simulink model "raised_cosine_filter"  (R2026a)
settings: Solver=VariableStepAuto
libraries: dsphdlsigops2 x2, simulink x1, hdlsllib x1

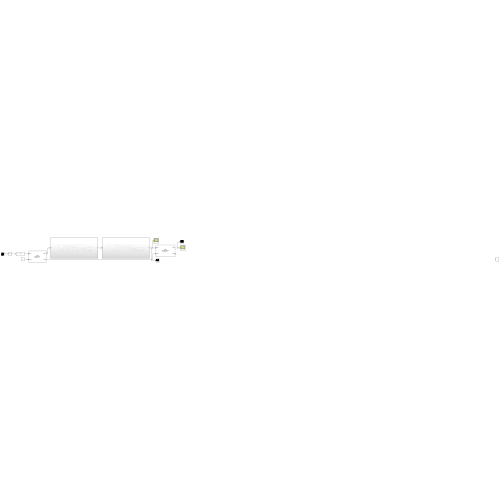
[thumbnail: Simulink's stored preview of the top-level diagram]
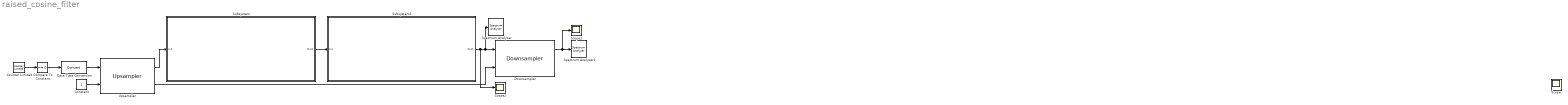
== system raised_cosine_filter ==
  Compare To Constant : simulink/Logic and Bit Operations/Compare To Constant  relop===  const=0  OutDataTypeStr=boolean
  Constant : Constant  OutDataTypeStr=boolean
  Counter Limited : hdlsllib/Sources/Counter Limited  uplimit=1000  tsamp=-1
  Data Type Conversion : DataTypeConversion  SaturateOnIntegerOverflow=off  RndMeth=Floor
  Downsampler : dsphdlsigops2/Downsampler  DownsampleFactor=4  SampleOffset=0  SimulateUsing=Code generation  ResetInputPort=off
  Scope : Scope
      settings: DataLoggingVariableName=ScopeData2  DataLoggingSaveFormat=Array
  Scope1 : Scope
      settings: ActiveDisplayYMinimum=-0.066624588581400856  ActiveDisplayYMaximum=0.22900316407454813  DataLoggingSaveFormat=Array
  Scope2 : Scope
      settings: ActiveDisplayYMinimum=-0.0763979925  ActiveDisplayYMaximum=0.2506889325  DataLoggingSaveFormat=Array
  Spectrum Analyzer : SpectrumAnalyzer  WindowPosition=[269.000000,92.000000,666.000000,500.000000,]  ScopeFrameLocation=window  WindowInvariantSamplesPerUpdate=on  YLimits=[-113.5521 -5.3787]
  Spectrum Analyzer1 : SpectrumAnalyzer  WindowPosition=[339.000000,58.000000,818.000000,500.000000,]  ScopeFrameLocation=window  WindowInvariantSamplesPerUpdate=on  YLimits=[-101.5109 6.6625]
  Subsystem : Subsystem
  Subsystem1 : Subsystem
  Upsampler : dsphdlsigops2/Upsampler  UpsampleFactor=4  SampleOffset=0  NumCycles=1  SimulateUsing=Code generation  ResetInputPort=off  ReadyPort=off
  wires:
  Downsampler/1 -> Scope1/1, Spectrum Analyzer1/1
  Subsystem1/1(Out1) -> Downsampler/1, Spectrum Analyzer/1, Scope2/1
  Upsampler/2 -> Downsampler/2
  Subsystem/1(Out1) -> Subsystem1/1(In1)
  Upsampler/1 -> Subsystem/1(In1)
  Constant/1 -> Upsampler/2
  Data Type Conversion/1 -> Upsampler/1
  Compare To Constant/1 -> Data Type Conversion/1
  Counter Limited/1 -> Compare To Constant/1

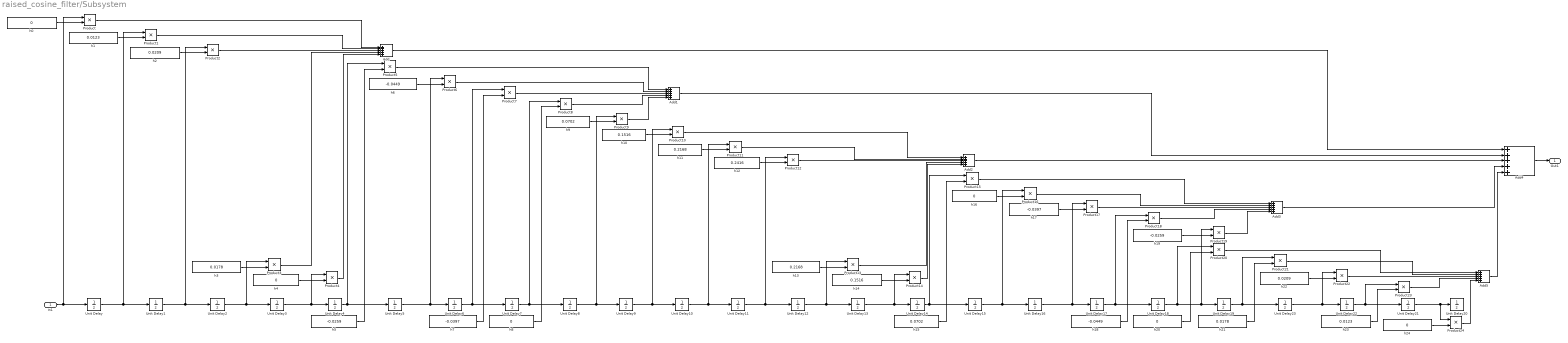
== system raised_cosine_filter/Subsystem ==
  In1 : Inport
  Add{,1..5} (6 alike) : Sum  Inputs=+++++
  Product{,1..24} (25 alike) : Product
  Unit Delay{,1..23} (24 alike) : UnitDelay  SampleTime=-1
  h{0,4,8,16,20,24} (6 alike) : Constant  Value=0
  h1 : Constant  Value=0.0123
  h10 : Constant  Value=0.1516
  h11 : Constant  Value=0.2168
  h12 : Constant  Value=0.2416
  h13 : Constant  Value=0.2168
  h14 : Constant  Value=0.1516
  h15 : Constant  Value=0.0702
  h17 : Constant  Value=-0.0397
  h18 : Constant  Value=-0.0449
  h19 : Constant  Value=-0.0259
  h2 : Constant  Value=0.0209
  h21 : Constant  Value=0.0178
  h22 : Constant  Value=0.0209
  h23 : Constant  Value=0.0123
  h3 : Constant  Value=0.0178
  h5 : Constant  Value=-0.0259
  h6 : Constant  Value=-0.0449
  h7 : Constant  Value=-0.0397
  h9 : Constant  Value=0.0702
  Out1 : Outport
  wires:
  Add4/1 -> Out1/1
  Add5/1 -> Add4/5
  Product24/1 -> Add5/5
  h24/1 -> Product24/2
  Unit Delay21/1 -> Product24/1, Unit Delay20/1
  Product23/1 -> Add5/4
  h23/1 -> Product23/2
  Unit Delay22/1 -> Unit Delay21/1, Product23/1
  Product22/1 -> Add5/3
  Unit Delay23/1 -> Product22/1, Unit Delay22/1
  h22/1 -> Product22/2
  Product21/1 -> Add5/2
  Product20/1 -> Add5/1
  Product19/1 -> Add3/5
  h20/1 -> Product20/2
  Unit Delay18/1 -> Product19/1, Unit Delay19/1, Product20/1
  Product18/1 -> Add3/4
  h19/1 -> Product19/2
  h9/1 -> Product9/2
  h8/1 -> Product8/2
  Product13/1 -> Add2/4
  Product6/1 -> Add1/2
  Unit Delay19/1 -> Product21/1, Unit Delay23/1
  h7/1 -> Product7/2
  Unit Delay6/1 -> Unit Delay7/1, Product7/1
  h12/1 -> Product12/2
  h6/1 -> Product6/2
  Unit Delay/1 -> Product1/1, Unit Delay1/1
  Unit Delay4/1 -> Product5/1, Unit Delay5/1
  Product4/1 -> Add/5
  Add1/1 -> Add4/2
  In1/1 -> Unit Delay/1, Product/1
  h1/1 -> Product1/2
  Product/1 -> Add/1
  Unit Delay11/1 -> Unit Delay12/1, Product12/1
  Unit Delay5/1 -> Product6/1, Unit Delay6/1
  Product11/1 -> Add2/2
  Product5/1 -> Add1/1
  h10/1 -> Product10/2
  h3/1 -> Product3/2
  Unit Delay16/1 -> Unit Delay17/1, Product17/1
  Product1/1 -> Add/2
  h13/1 -> Product13/2
  Product2/1 -> Add/3
  h0/1 -> Product/2
  Product3/1 -> Add/4
  Product8/1 -> Add1/4
  Add/1 -> Add4/1
  Add3/1 -> Add4/4
  Unit Delay3/1 -> Unit Delay4/1, Product4/1
  Unit Delay2/1 -> Product3/1, Unit Delay3/1
  h5/1 -> Product5/2
  h4/1 -> Product4/2
  h17/1 -> Product17/2
  Unit Delay8/1 -> Unit Delay9/1, Product9/1
  h11/1 -> Product11/2
  Unit Delay15/1 -> Product16/1, Unit Delay16/1
  h2/1 -> Product2/2
  Product9/1 -> Add1/5
  Unit Delay9/1 -> Product10/1, Unit Delay10/1
  Product15/1 -> Add3/1
  Product10/1 -> Add2/1
  Product12/1 -> Add2/3
  Unit Delay13/1 -> Unit Delay14/1, Product14/1
  Unit Delay10/1 -> Unit Delay11/1, Product11/1
  Unit Delay12/1 -> Product13/1, Unit Delay13/1
  h14/1 -> Product14/2
  Product14/1 -> Add2/5
  Product7/1 -> Add1/3
  Unit Delay14/1 -> Product15/1, Unit Delay15/1
  h15/1 -> Product15/2
  Unit Delay7/1 -> Product8/1, Unit Delay8/1
  Add2/1 -> Add4/3
  h16/1 -> Product16/2
  h21/1 -> Product21/2
  Product16/1 -> Add3/2
  Product17/1 -> Add3/3
  Unit Delay1/1 -> Product2/1, Unit Delay2/1
  Unit Delay17/1 -> Unit Delay18/1, Product18/1
  h18/1 -> Product18/2

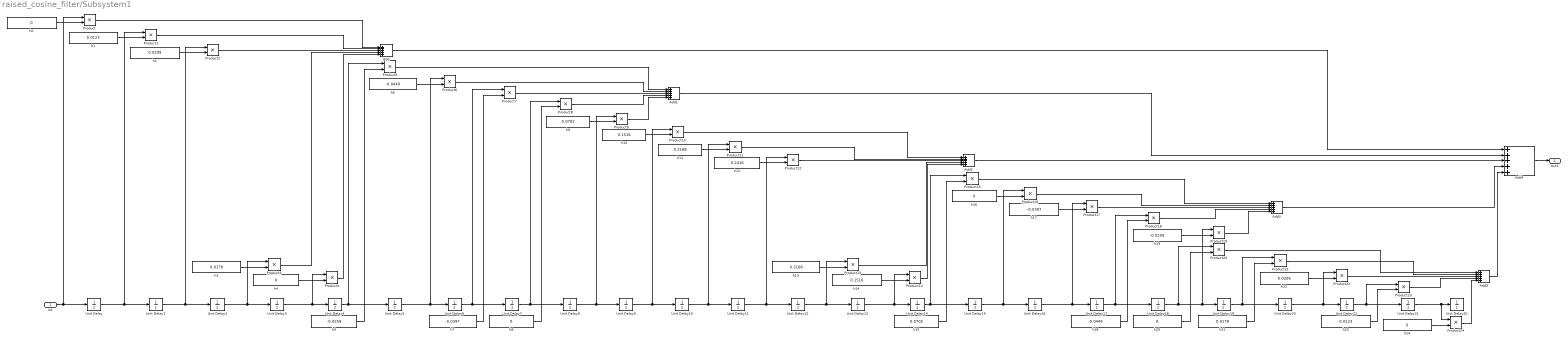
== system raised_cosine_filter/Subsystem1 ==
  In1 : Inport
  Add{,1..5} (6 alike) : Sum  Inputs=+++++
  Product{,1..24} (25 alike) : Product
  Unit Delay{,1..23} (24 alike) : UnitDelay  SampleTime=-1
  h{0,4,8,16,20,24} (6 alike) : Constant  Value=0
  h1 : Constant  Value=0.0123
  h10 : Constant  Value=0.1516
  h11 : Constant  Value=0.2168
  h12 : Constant  Value=0.2416
  h13 : Constant  Value=0.2168
  h14 : Constant  Value=0.1516
  h15 : Constant  Value=0.0702
  h17 : Constant  Value=-0.0397
  h18 : Constant  Value=-0.0449
  h19 : Constant  Value=-0.0259
  h2 : Constant  Value=0.0209
  h21 : Constant  Value=0.0178
  h22 : Constant  Value=0.0209
  h23 : Constant  Value=0.0123
  h3 : Constant  Value=0.0178
  h5 : Constant  Value=-0.0259
  h6 : Constant  Value=-0.0449
  h7 : Constant  Value=-0.0397
  h9 : Constant  Value=0.0702
  Out1 : Outport
  wires:
  Add4/1 -> Out1/1
  Add5/1 -> Add4/5
  Product24/1 -> Add5/5
  h24/1 -> Product24/2
  Unit Delay21/1 -> Product24/1, Unit Delay20/1
  Product23/1 -> Add5/4
  h23/1 -> Product23/2
  Unit Delay22/1 -> Unit Delay21/1, Product23/1
  Product22/1 -> Add5/3
  Unit Delay23/1 -> Product22/1, Unit Delay22/1
  h22/1 -> Product22/2
  Product21/1 -> Add5/2
  Product20/1 -> Add5/1
  Product19/1 -> Add3/5
  h20/1 -> Product20/2
  Unit Delay18/1 -> Product19/1, Unit Delay19/1, Product20/1
  Product18/1 -> Add3/4
  h19/1 -> Product19/2
  h9/1 -> Product9/2
  h8/1 -> Product8/2
  Product13/1 -> Add2/4
  Product6/1 -> Add1/2
  Unit Delay19/1 -> Product21/1, Unit Delay23/1
  h7/1 -> Product7/2
  Unit Delay6/1 -> Unit Delay7/1, Product7/1
  h12/1 -> Product12/2
  h6/1 -> Product6/2
  Unit Delay/1 -> Product1/1, Unit Delay1/1
  Unit Delay4/1 -> Product5/1, Unit Delay5/1
  Product4/1 -> Add/5
  Add1/1 -> Add4/2
  In1/1 -> Unit Delay/1, Product/1
  h1/1 -> Product1/2
  Product/1 -> Add/1
  Unit Delay11/1 -> Unit Delay12/1, Product12/1
  Unit Delay5/1 -> Product6/1, Unit Delay6/1
  Product11/1 -> Add2/2
  Product5/1 -> Add1/1
  h10/1 -> Product10/2
  h3/1 -> Product3/2
  Unit Delay16/1 -> Unit Delay17/1, Product17/1
  Product1/1 -> Add/2
  h13/1 -> Product13/2
  Product2/1 -> Add/3
  h0/1 -> Product/2
  Product3/1 -> Add/4
  Product8/1 -> Add1/4
  Add/1 -> Add4/1
  Add3/1 -> Add4/4
  Unit Delay3/1 -> Unit Delay4/1, Product4/1
  Unit Delay2/1 -> Product3/1, Unit Delay3/1
  h5/1 -> Product5/2
  h4/1 -> Product4/2
  h17/1 -> Product17/2
  Unit Delay8/1 -> Unit Delay9/1, Product9/1
  h11/1 -> Product11/2
  Unit Delay15/1 -> Product16/1, Unit Delay16/1
  h2/1 -> Product2/2
  Product9/1 -> Add1/5
  Unit Delay9/1 -> Product10/1, Unit Delay10/1
  Product15/1 -> Add3/1
  Product10/1 -> Add2/1
  Product12/1 -> Add2/3
  Unit Delay13/1 -> Unit Delay14/1, Product14/1
  Unit Delay10/1 -> Unit Delay11/1, Product11/1
  Unit Delay12/1 -> Product13/1, Unit Delay13/1
  h14/1 -> Product14/2
  Product14/1 -> Add2/5
  Product7/1 -> Add1/3
  Unit Delay14/1 -> Product15/1, Unit Delay15/1
  h15/1 -> Product15/2
  Unit Delay7/1 -> Product8/1, Unit Delay8/1
  Add2/1 -> Add4/3
  h16/1 -> Product16/2
  h21/1 -> Product21/2
  Product16/1 -> Add3/2
  Product17/1 -> Add3/3
  Unit Delay1/1 -> Product2/1, Unit Delay2/1
  Unit Delay17/1 -> Unit Delay18/1, Product18/1
  h18/1 -> Product18/2
